simulink subsystem "PVcontroller"  (R2023a)
settings: Solver=VariableStepAuto  StartTime=0.0  StopTime=10.0  RelTol=1e-3
model mask{L=PVInverter.L, frequency=Grid.frequency, iMax=PVInverter.I_max_pu, zBase=Base.z_base, mVAbase=Base.MVA_base_new, VdcBase=PVController.Vdc_base, sampleTime=-1, Choice=Incremental conductance (INC), Vdc=PVInverter.Vdc, delV=10, tSettling=Mpp.ts, Kppll=PLL.Kp_pll, Kipll=PLL.Ki_pll, initialPhase=0, Kpv=PVController.Kp_v, Kiv=PVController.Ki_v, Kdv=0, Kpicd=PVController.Kp_ic, Kiicd=PVController.Ki_ic, Kdicd=0, Kpicq=PVController.Kp_ic, Kiicq=PVController.Ki_ic, Kdicq=0}
  mask prompts: L "AC Filter Inductance (H)"; frequency "System Frequency (Hz)"; iMax "Inverter Current Limit (PU)"; zBase "Base Impedance AC Side (Ohm)"; mVAbase "Base  Volt Amper AC side"; VdcBase "DC Bus Base Voltage (V)"; Choice "Algorithm"; Vdc "Initial VoltageFor MPPT"; delV "Voltage StepOf MPPT"; tSettling "Settling Time Of MPPT (s)"; Kppll "Proportional Gain"; Kipll "Integral Gain"; initialPhase "Initial phase angle (deg)"; Kpv "Proportional Gain"; Kiv "Integral Gain"; Kdv "Derivative Gain"; Kpicd "Daxis Proportional Gain"; Kiicd "Daxis Integral Gain"; Kdicd "D axis Derivative Gain"; Kpicq "Q axis Proportional Gain"; Kiicq "Qaxis Integral Gain"; Kdicq "Qaxis Derivative Gain"
undefined symbols (not defined in the file): Mpp, Ts
libraries: simulink x10, eeGeneralControl x4, slpidlib x3, eeTransforms x3, eeSinusoidalMeasurementV2 x1
settings Model: Creator=rajarshd  LastModifiedBy=Rajarshi

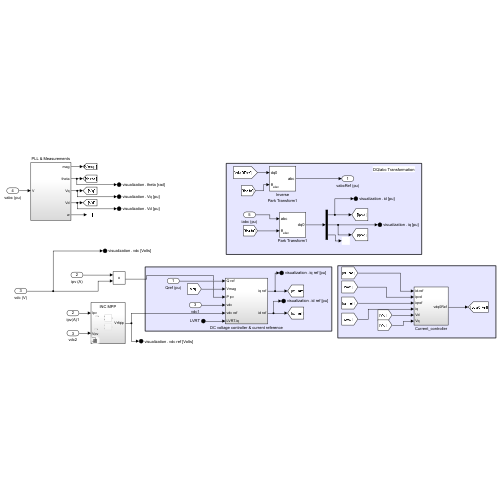
[thumbnail: Simulink's stored preview of the top-level diagram]
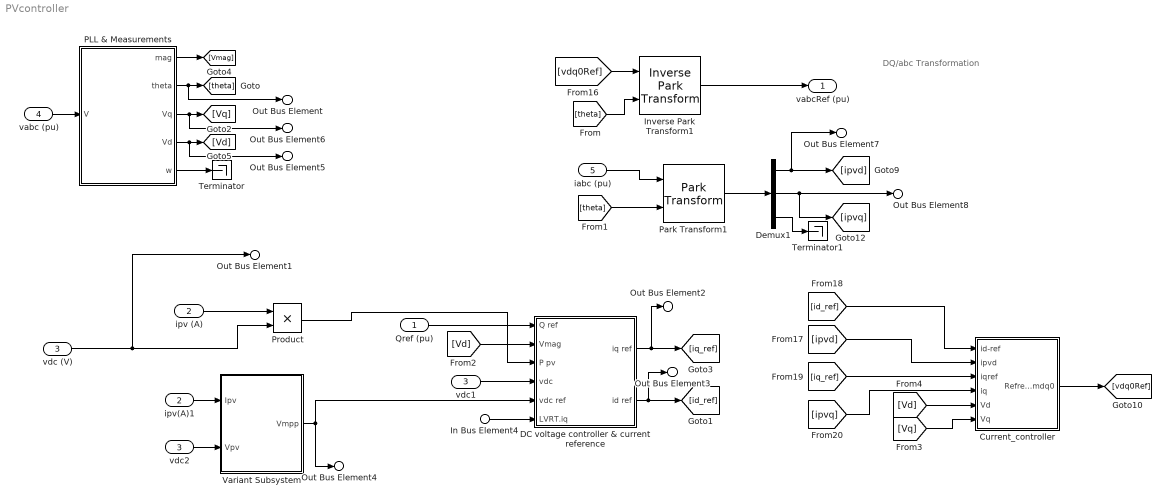
== system PVcontroller ==
  note: DQ/abc Transformation
  Qref (pu) : Inport
  ipv (A) : Inport  Port=2
  vdc (V) : Inport  Port=3
  vabc (pu) : Inport  Port=4
  iabc (pu) : Inport  Port=5
  In Bus Element4 : Inport  Port=6  PortName=LVRT
  Current_controller : Subsystem  SystemSampleTime=sampleTime
  DC voltage controller & current reference : Subsystem  SystemSampleTime=sampleTime
  Demux1 : Demux  Outputs=3
  Inverse Park Transform1 : eeTransforms/Inverse Park Transform  AxisAlignment=Q-axis  PowerInvariant=off
  PLL & Measurements : Subsystem
      settings: PortSchema="{\"entries\":[{\"content\":{\"sides\":[{\"content\":{\"connectorIds\":[\"Out1\",\"Out2\",\"Out3\",\"Out4\",\"Out5\"]},\"type\":\"ConnectorPlacement.EquallySpacedRectSide\",\"uuid\":\"76485780-20fe-4fcf-8224-69648da6ed2a\"},{\"content\":{\"connectorIds\":[\"In1\"],\"side\":\"RIGHT\"},\"type\":\"ConnectorPlacement.EquallySpacedRectSide\",\"uuid\":\"f19a6390-e634-42c7-8d46-4cd80cbab182\"},{\"content\":{\"side\":\"TOP\"},\"type\":\"ConnectorPlacement.EquallySpacedRectSide\",\"uuid\":\"87682f72-1844-428e-be70-ad7ca3191ee3\"}]},\"type\":\"ConnectorPlacement.EquallySpacedConnector\",\"uuid\":\"f2136b07-48ec-402b-adb3-18c0bac2157c\"}],\"packageUris\":[\"http://schema.mathworks.com/mf0/Connector/R2020b\"],\"version\":\"1.0\"}"
  Park Transform1 : eeTransforms/Park Transform  AxisAlignment=Q-axis  PowerInvariant=off
  Product : Product
  Terminator : Terminator
  Terminator1 : Terminator
  Variant Subsystem : Subsystem  Variant=on  VariantControlMode=label  LabelModeActiveChoice=Incremental conductance (INC)
  ipv(A)1 : InportShadow  Port=2
  vdc1 : InportShadow  Port=3
  vdc2 : InportShadow  Port=3
  vabcRef (pu) : Outport
  Out Bus Element : Outport  Port=2  PortName=visualization  Element=theta [rad]
  Out Bus Element1 : Outport  Port=2  PortName=visualization  Element=vdc [Volts]
  Out Bus Element2 : Outport  Port=2  PortName=visualization  Element=iq ref [pu]
  Out Bus Element3 : Outport  Port=2  PortName=visualization  Element=id ref [pu]
  Out Bus Element4 : Outport  Port=2  PortName=visualization  Element=vdc ref [Volts]
  Out Bus Element5 : Outport  Port=2  PortName=visualization  Element=Vd [pu]
  Out Bus Element6 : Outport  Port=2  PortName=visualization  Element=Vq [pu]
  Out Bus Element7 : Outport  Port=2  PortName=visualization  Element=id [pu]
  Out Bus Element8 : Outport  Port=2  PortName=visualization  Element=iq [pu]
  wires:
  PLL & Measurements/2(theta) -> Out Bus Element/1, [theta]
  ipv(A)1/1 -> Variant Subsystem/1(Ipv)
  vdc2/1 -> Variant Subsystem/2(Vpv)
  ipv (A)/1 -> Product/1
  PLL & Measurements/5(w) -> Terminator/1
  Variant Subsystem/1(Vmpp) -> Out Bus Element4/1, DC voltage controller & current reference/5(vdc ref)
  vdc1/1 -> DC voltage controller & current reference/4(vdc)
  vabc (pu)/1 -> PLL & Measurements/1(V)
  PLL & Measurements/4(Vd) -> Out Bus Element5/1, [Vd]
  PLL & Measurements/1(mag) -> [Vmag]
  PLL & Measurements/3(Vq) -> Out Bus Element6/1, [Vq]
  Product/1 -> DC voltage controller & current reference/3(P pv)
  vdc (V)/1 -> Out Bus Element1/1, Product/2
  Qref (pu)/1 -> DC voltage controller & current reference/1(Q ref)
  DC voltage controller & current reference/2(id ref) -> Out Bus Element3/1, [id_ref]
  DC voltage controller & current reference/1(iq ref) -> Out Bus Element2/1, [iq_ref]
  [Vd] -> DC voltage controller & current reference/2(Vmag)
  iabc (pu)/1 -> Park Transform1/1
  [ipvd] -> Current_controller/2(ipvd)
  [theta] -> Inverse Park Transform1/2
  [theta] -> Park Transform1/2
  [ipvq] -> Current_controller/4(iq)
  [iq_ref] -> Current_controller/3(iqref)
  [Vd] -> Current_controller/5(Vd)
  [id_ref] -> Current_controller/1(id-ref)
  Park Transform1/1 -> Demux1/1
  [vdq0Ref] -> Inverse Park Transform1/1
  Demux1/3 -> Terminator1/1
  Demux1/1 -> Out Bus Element7/1, [ipvd]
  Inverse Park Transform1/1 -> vabcRef (pu)/1
  Demux1/2 -> Out Bus Element8/1, [ipvq]
  Current_controller/1(Refrence_mdq0) -> [vdq0Ref]
  [Vq] -> Current_controller/6(Vq)
  In Bus Element4/1 -> DC voltage controller & current reference/6(LVRT.iq)

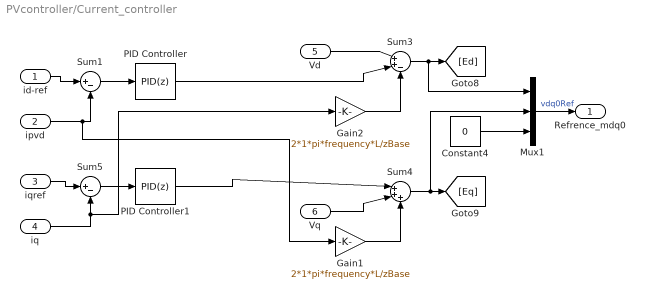
== system PVcontroller/Current_controller ==
  id-ref : Inport
  ipvd : Inport  Port=2
  iqref : Inport  Port=3
  iq : Inport  Port=4
  Vd : Inport  Port=5
  Vq : Inport  Port=6
  Constant4 : Constant  Value=0
  Gain1 : Gain  Gain=2*1*pi*frequency*L/zBase
  Gain2 : Gain  Gain=2*1*pi*frequency*L/zBase
  Mux1 : Mux  Inputs=3
  PID Controller : slpidlib/PID Controller  Controller=PID  Form=Parallel  TimeDomain=Discrete-time  UseExternalTs=off  SampleTime=-1  IntegratorMethod=Forward Euler  FilterMethod=Forward Euler  ControllerParametersSource=internal  P=Kpicd  I=Kiicd  UseKiTs=off  D=Kdicd  N=100  UseFilter=on  TunerSelectOption=Transfer Function Based (PID Tuner App)  InitialConditionSource=internal  InitialConditionForIntegrator=0  InitialConditionForFilter=0  DifferentiatorICPrevScaledInput=0  ExternalReset=none  TrackingMode=off  Kt=1  LimitOutput=off  SatLimitsSource=internal  UpperSaturationLimit=inf  LowerSaturationLimit=-inf  LinearizeAsGain=on  AntiWindupMode=clamping  Kb=1  LimitIntegrator=off  UpperIntegratorSaturationLimit=inf  LowerIntegratorSaturationLimit=-inf  POutMin=[]  POutMax=[]  IOutMin=[]  IOutMax=[]  DOutMin=[]  DOutMax=[]  NOutMin=[]  NOutMax=[]  SumOutMin=[]  SumOutMax=[]  SaturationOutMin=[]  SaturationOutMax=[]  PParamMin=[]  PParamMax=[]  IParamMin=[]  IParamMax=[]  DParamMin=[]  DParamMax=[]  NParamMin=[]  NParamMax=[]  KbParamMin=[]  KbParamMax=[]  KtParamMin=[]  KtParamMax=[]  KbOutMin=[]  KbOutMax=[]  KtOutMin=[]  KtOutMax=[]  IntegratorOutMin=[]  IntegratorOutMax=[]  FilterOutMin=[]  FilterOutMax=[]  SumI1OutMin=[]  SumI1OutMax=[]  SumI2OutMin=[]  SumI2OutMax=[]  SumI3OutMin=[]  SumI3OutMax=[]  SumI4OutMin=[]  SumI4OutMax=[]  SumDOutMin=[]  SumDOutMax=[]  DifferentiatorOutMin=[]  DifferentiatorOutMax=[]  FilterDiffOutCoefMin=[]  FilterDiffOutCoefMax=[]  ReciprocalOutMin=[]  ReciprocalOutMax=[]  SumDenOutMin=[]  SumDenOutMax=[]  SumNumOutMin=[]  SumNumOutMax=[]  DivideOutMin=[]  DivideOutMax=[]  UdiffTsProdOutMin=[]  UdiffTsProdOutMax=[]  NTsProdOutMin=[]  NTsProdOutMax=[]  UintegralTsProdOutMin=[]  UintegralTsProdOutMax=[]  UngainTsProdOutMin=[]  UngainTsProdOutMax=[]  ClampingZeroOutDataTypeStr=Inherit: Inherit via back propagation  ClampingZeroOutMin=[]  ClampingZeroOutMax=[]  FilterDenConstantOutDataTypeStr=Inherit: Inherit via back propagation  FilterDenConstantOutMin=[]  FilterDenConstantOutMax=[]  PCopyOutDataTypeStr=Inherit: Inherit via back propagation  PCopyOutMin=[]  PCopyOutMax=[]  NCopyOutDataTypeStr=Inherit: Inherit via back propagation  NCopyOutMin=[]  NCopyOutMax=[]  IntegratorContinuousStateAttributes=''  IntegratorStateMustResolveToSignalObject=off  IntegratorRTWStateStorageClass=Auto  FilterContinuousStateAttributes=''  FilterStateMustResolveToSignalObject=off  FilterRTWStateStorageClass=Auto  ParallelPVariant=InternalParameters  IdealPVariant=Disabled  IVariant=InternalParameters  DVariant=InternalParameters  IntegratorVariant=Discrete  SatVariant=Disabled  AWVariant=Passthrough  PCopyVariant=Disabled  TRVariant=Disabled  FdbkBlocksVariant=Forward  IdealPFdbkVariant=Disabled  SatFdbkVariant=Disabled  DerivativeFilterVariant=ForwardEulerFilter  NVariant=InternalParameters  NCopyVariant=Disabled  FilterICVariant=InternalICsFilter  IntegratorICVariant=InternalICs  ExternalResetVariant=Disabled  TRSumVariant=Passthrough  SumFdbkVariant=Disabled  SumVariant=Sum_PID  TsampFilterVariant=InternalTs  TsampNgainVariant=Passthrough  TsampIntegralVariant=Disabled_SignalSpec  ExternalSaturationOutDataTypeStr=Inherit: Same as second input
  PID Controller1 : slpidlib/PID Controller  Controller=PID  Form=Parallel  TimeDomain=Discrete-time  UseExternalTs=off  SampleTime=-1  IntegratorMethod=Forward Euler  FilterMethod=Forward Euler  ControllerParametersSource=internal  P=Kpicq  I=Kiicq  UseKiTs=off  D=Kdicq  N=100  UseFilter=on  TunerSelectOption=Transfer Function Based (PID Tuner App)  InitialConditionSource=internal  InitialConditionForIntegrator=0  InitialConditionForFilter=0  DifferentiatorICPrevScaledInput=0  ExternalReset=none  TrackingMode=off  Kt=1  LimitOutput=off  SatLimitsSource=internal  UpperSaturationLimit=inf  LowerSaturationLimit=-inf  LinearizeAsGain=on  AntiWindupMode=none  Kb=1  LimitIntegrator=off  UpperIntegratorSaturationLimit=inf  LowerIntegratorSaturationLimit=-inf  POutMin=[]  POutMax=[]  IOutMin=[]  IOutMax=[]  DOutMin=[]  DOutMax=[]  NOutMin=[]  NOutMax=[]  SumOutMin=[]  SumOutMax=[]  SaturationOutMin=[]  SaturationOutMax=[]  PParamMin=[]  PParamMax=[]  IParamMin=[]  IParamMax=[]  DParamMin=[]  DParamMax=[]  NParamMin=[]  NParamMax=[]  KbParamMin=[]  KbParamMax=[]  KtParamMin=[]  KtParamMax=[]  KbOutMin=[]  KbOutMax=[]  KtOutMin=[]  KtOutMax=[]  IntegratorOutMin=[]  IntegratorOutMax=[]  FilterOutMin=[]  FilterOutMax=[]  SumI1OutMin=[]  SumI1OutMax=[]  SumI2OutMin=[]  SumI2OutMax=[]  SumI3OutMin=[]  SumI3OutMax=[]  SumI4OutMin=[]  SumI4OutMax=[]  SumDOutMin=[]  SumDOutMax=[]  DifferentiatorOutMin=[]  DifferentiatorOutMax=[]  FilterDiffOutCoefMin=[]  FilterDiffOutCoefMax=[]  ReciprocalOutMin=[]  ReciprocalOutMax=[]  SumDenOutMin=[]  SumDenOutMax=[]  SumNumOutMin=[]  SumNumOutMax=[]  DivideOutMin=[]  DivideOutMax=[]  UdiffTsProdOutMin=[]  UdiffTsProdOutMax=[]  NTsProdOutMin=[]  NTsProdOutMax=[]  UintegralTsProdOutMin=[]  UintegralTsProdOutMax=[]  UngainTsProdOutMin=[]  UngainTsProdOutMax=[]  ClampingZeroOutDataTypeStr=Inherit: Inherit via back propagation  ClampingZeroOutMin=[]  ClampingZeroOutMax=[]  FilterDenConstantOutDataTypeStr=Inherit: Inherit via back propagation  FilterDenConstantOutMin=[]  FilterDenConstantOutMax=[]  PCopyOutDataTypeStr=Inherit: Inherit via back propagation  PCopyOutMin=[]  PCopyOutMax=[]  NCopyOutDataTypeStr=Inherit: Inherit via back propagation  NCopyOutMin=[]  NCopyOutMax=[]  IntegratorContinuousStateAttributes=''  IntegratorStateMustResolveToSignalObject=off  IntegratorRTWStateStorageClass=Auto  FilterContinuousStateAttributes=''  FilterStateMustResolveToSignalObject=off  FilterRTWStateStorageClass=Auto  ParallelPVariant=InternalParameters  IdealPVariant=Disabled  IVariant=InternalParameters  DVariant=InternalParameters  IntegratorVariant=Discrete  SatVariant=Disabled  AWVariant=Passthrough  PCopyVariant=Disabled  TRVariant=Disabled  FdbkBlocksVariant=Forward  IdealPFdbkVariant=Disabled  SatFdbkVariant=Disabled  DerivativeFilterVariant=ForwardEulerFilter  NVariant=InternalParameters  NCopyVariant=Disabled  FilterICVariant=InternalICsFilter  IntegratorICVariant=InternalICs  ExternalResetVariant=Disabled  TRSumVariant=Passthrough  SumFdbkVariant=Disabled  SumVariant=Sum_PID  TsampFilterVariant=InternalTs  TsampNgainVariant=Passthrough  TsampIntegralVariant=Disabled_SignalSpec  ExternalSaturationOutDataTypeStr=Inherit: Same as second input
  Sum1 : Sum  Inputs=|+-
  Sum3 : Sum  Inputs=|++-
  Sum4 : Sum  Inputs=|+++
  Sum5 : Sum  Inputs=|+-
  Refrence_mdq0 : Outport
  wires:
  PID Controller/1 -> Sum3/2
  Sum3/1 -> Mux1/1, [Ed]
  Gain2/1 -> Sum3/3
  ipvd/1 -> Gain1/1, Sum1/2
  id-ref/1 -> Sum1/1
  Gain1/1 -> Sum4/3
  Vq/1 -> Sum4/2
  iq/1 -> Gain2/1, Sum5/2
  Sum1/1 -> PID Controller/1
  Vd/1 -> Sum3/1
  Constant4/1 -> Mux1/3
  Sum5/1 -> PID Controller1/1
  iqref/1 -> Sum5/1
  PID Controller1/1 -> Sum4/1
  Sum4/1 -> Mux1/2, [Eq]
  Mux1/1 -> Refrence_mdq0/1  "vdq0Ref"

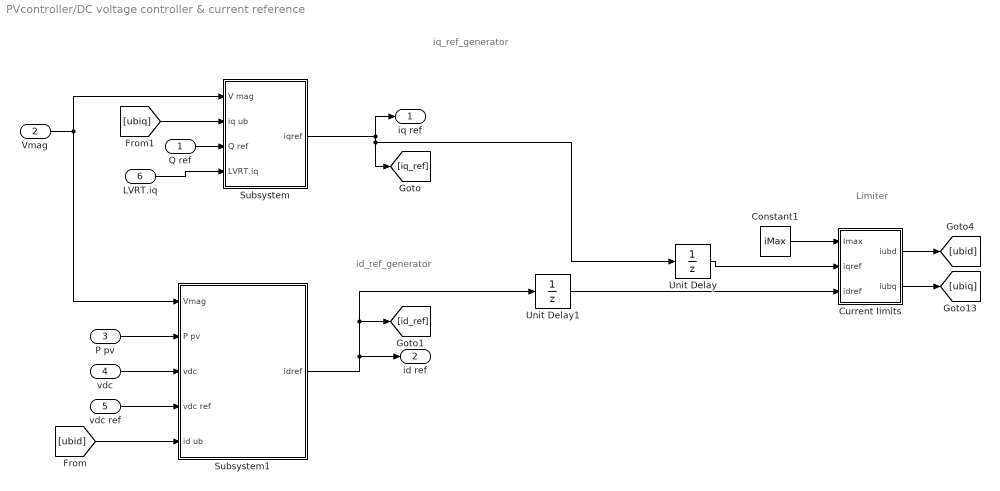
== system PVcontroller/DC voltage controller & current reference ==
  note: Limiter
  note: iq_ref_generator
  note: id_ref_generator
  Q ref : Inport
  Vmag : Inport  Port=2
  P pv : Inport  Port=3
  vdc : Inport  Port=4
  vdc ref : Inport  Port=5
  LVRT.iq : Inport  Port=6
  Constant1 : Constant  Value=iMax
  Current limits : Subsystem
  Subsystem : Subsystem
  Subsystem1 : Subsystem
  Unit Delay : UnitDelay  SampleTime=-1  HasFrameUpgradeWarning=on
  Unit Delay1 : UnitDelay  SampleTime=-1  HasFrameUpgradeWarning=on
  iq ref : Outport
  id ref : Outport  Port=2
  wires:
  Unit Delay1/1 -> Current limits/3(idref)
  Unit Delay/1 -> Current limits/2(iqref)
  LVRT.iq/1 -> Subsystem/4(LVRT.iq)
  Current limits/2(iubq) -> [ubiq]
  Current limits/1(iubd) -> [ubid]
  Constant1/1 -> Current limits/1(Imax)
  Q ref/1 -> Subsystem/3(Q ref)
  Subsystem1/1(idref) -> [id_ref], Unit Delay1/1, id ref/1
  P pv/1 -> Subsystem1/2(P pv)
  vdc/1 -> Subsystem1/3(vdc)
  vdc ref/1 -> Subsystem1/4(vdc ref)
  Subsystem/1(iqref) -> Unit Delay/1, [iq_ref], iq ref/1
  [ubid] -> Subsystem1/5(id ub)
  [ubiq] -> Subsystem/2(iq ub)
  Vmag/1 -> Subsystem1/1(Vmag), Subsystem/1(V mag)

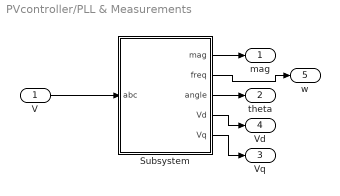
== system PVcontroller/PLL & Measurements ==
  V : Inport
  Subsystem : Subsystem
  mag : Outport
  theta : Outport  Port=2
  Vq : Outport  Port=3
  Vd : Outport  Port=4
  w : Outport  Port=5
  wires:
  V/1 -> Subsystem/1(abc)
  Subsystem/1(mag) -> mag/1
  Subsystem/3(angle) -> theta/1
  Subsystem/5(Vq) -> Vq/1
  Subsystem/4(Vd) -> Vd/1
  Subsystem/2(freq) -> w/1

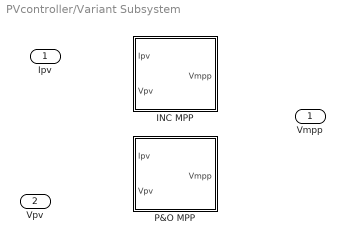
== system PVcontroller/Variant Subsystem ==
  Ipv : Inport
  Vpv : Inport  Port=2
  INC MPP : Subsystem  VariantControl=Incremental conductance (INC)
  P&O MPP : Subsystem  VariantControl=Perturb and observe (P&O)
  Vmpp : Outport

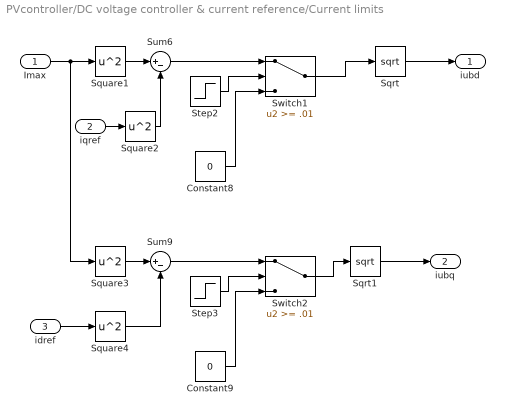
== system PVcontroller/DC voltage controller & current reference/Current limits ==
  Imax : Inport
  iqref : Inport  Port=2
  idref : Inport  Port=3
  Constant8 : Constant  Value=0
  Constant9 : Constant  Value=0
  Sqrt : Sqrt
  Sqrt1 : Sqrt
  Square{1..4} (4 alike) : Math  Operator=square
  Step2 : Step  Time=0.01  SampleTime=Ts
  Step3 : Step  Time=0.01  SampleTime=Ts
  Sum6 : Sum  Inputs=|+-
  Sum9 : Sum  Inputs=|+-
  Switch1 : Switch  Threshold=.01  SaturateOnIntegerOverflow=off  InputSameDT=off
  Switch2 : Switch  Threshold=.01  SaturateOnIntegerOverflow=off  InputSameDT=off
  iubd : Outport
  iubq : Outport  Port=2
  wires:
  idref/1 -> Square4/1
  Sqrt1/1 -> iubq/1
  Imax/1 -> Square1/1, Square3/1
  Sqrt/1 -> iubd/1
  Constant9/1 -> Switch2/3
  Square4/1 -> Sum9/2
  Constant8/1 -> Switch1/3
  Square2/1 -> Sum6/2
  Sum6/1 -> Switch1/1
  Square3/1 -> Sum9/1
  iqref/1 -> Square2/1
  Switch1/1 -> Sqrt/1
  Square1/1 -> Sum6/1
  Switch2/1 -> Sqrt1/1
  Step2/1 -> Switch1/2
  Step3/1 -> Switch2/2
  Sum9/1 -> Switch2/1

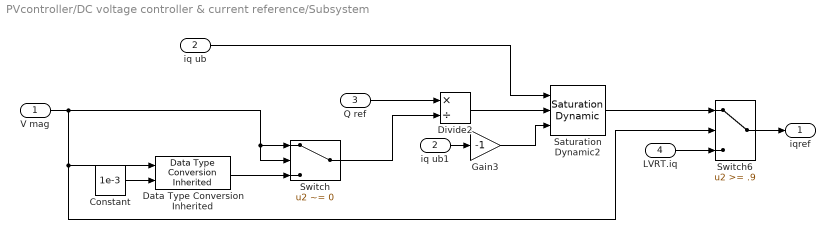
== system PVcontroller/DC voltage controller & current reference/Subsystem ==
  V mag : Inport
  iq ub : Inport  Port=2
  Q ref : Inport  Port=3
  LVRT.iq : Inport  Port=4
  Constant : Constant  Value=1e-3
  Data Type Conversion Inherited : simulink/Signal Attributes/Data Type Conversion Inherited  ConvertRealWorld=Real World Value  DoSatur=off
  Divide2 : Product  Inputs=*/
  Gain3 : Gain  Gain=-1
  Saturation Dynamic2 : simulink/Discontinuities/Saturation Dynamic  OutMin=[]  OutMax=[]  OutDataTypeStr=Inherit: Same as second input  OutDataType=fixdt(1, 16)  OutScaling=2^-10  DoSatur=off
  Switch : Switch  Criteria=u2 ~= 0  SaturateOnIntegerOverflow=off  InputSameDT=off
  Switch6 : Switch  Threshold=.9  SaturateOnIntegerOverflow=off  InputSameDT=off
  iq ub1 : InportShadow  Port=2
  iqref : Outport
  wires:
  LVRT.iq/1 -> Switch6/3
  Switch6/1 -> iqref/1
  Saturation Dynamic2/1 -> Switch6/1
  iq ub1/1 -> Gain3/1
  Divide2/1 -> Saturation Dynamic2/2
  Q ref/1 -> Divide2/1
  Gain3/1 -> Saturation Dynamic2/3
  iq ub/1 -> Saturation Dynamic2/1
  V mag/1 -> Switch/2, Switch/1, Switch6/2, Data Type Conversion Inherited/1
  Switch/1 -> Divide2/2
  Constant/1 -> Data Type Conversion Inherited/2
  Data Type Conversion Inherited/1 -> Switch/3

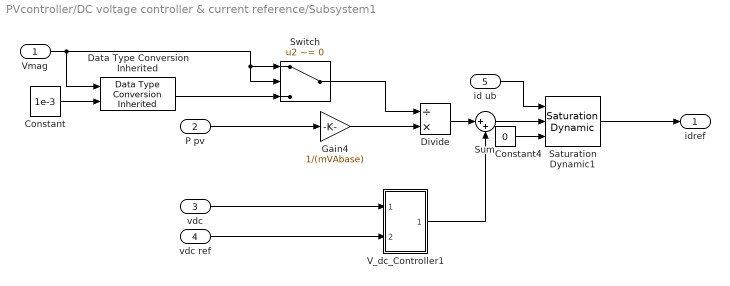
== system PVcontroller/DC voltage controller & current reference/Subsystem1 ==
  Vmag : Inport
  P pv : Inport  Port=2
  vdc : Inport  Port=3
  vdc ref : Inport  Port=4
  id ub : Inport  Port=5
  Constant : Constant  Value=1e-3
  Constant4 : Constant  Value=0
  Data Type Conversion Inherited : simulink/Signal Attributes/Data Type Conversion Inherited  ConvertRealWorld=Real World Value  DoSatur=off
  Divide : Product  Inputs=/*
  Gain4 : Gain  Gain=1/(mVAbase)
  Saturation Dynamic1 : simulink/Discontinuities/Saturation Dynamic  OutMin=[]  OutMax=[]  OutDataTypeStr=Inherit: Same as second input  OutDataType=fixdt(1, 16)  OutScaling=2^-10  DoSatur=off
  Sum : Sum  Inputs=|++
  Switch : Switch  Criteria=u2 ~= 0  SaturateOnIntegerOverflow=off  InputSameDT=off
  V_dc_Controller1 : Subsystem
  idref : Outport
  wires:
  Saturation Dynamic1/1 -> idref/1
  Constant4/1 -> Saturation Dynamic1/3
  P pv/1 -> Gain4/1
  V_dc_Controller1/1(Out1) -> Sum/2
  Sum/1 -> Saturation Dynamic1/2
  vdc ref/1 -> V_dc_Controller1/2(vdc ref)
  id ub/1 -> Saturation Dynamic1/1
  Gain4/1 -> Divide/2
  Divide/1 -> Sum/1
  vdc/1 -> V_dc_Controller1/1(vdc)
  Vmag/1 -> Data Type Conversion Inherited/1, Switch/2, Switch/1
  Switch/1 -> Divide/1
  Constant/1 -> Data Type Conversion Inherited/2
  Data Type Conversion Inherited/1 -> Switch/3

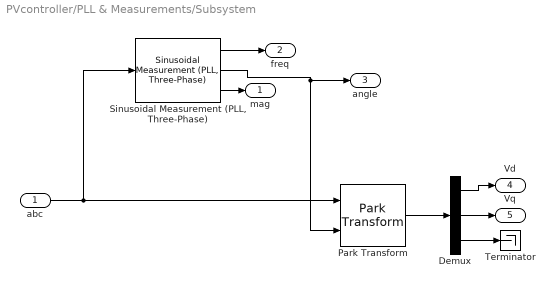
== system PVcontroller/PLL & Measurements/Subsystem ==
  abc : Inport
  Demux : Demux  Outputs=3
  Park Transform : eeTransforms/Park Transform  AxisAlignment=Q-axis  PowerInvariant=off
  "Sinusoidal Measurement (PLL, Three-Phase)" : eeSinusoidalMeasurementV2/Sinusoidal Measurement (PLL, Three-Phase)  Kp_LF=Kppll  Ki_LF=Kipll  F0=frequency  Theta0=initialPhase  Ts=sampleTime
      link override Park Transform: PowerInvariant=off
  Terminator : Terminator
  mag : Outport
  freq : Outport  Port=2
  angle : Outport  Port=3
  Vd : Outport  Port=4
  Vq : Outport  Port=5
  wires:
  Demux/3 -> Terminator/1
  abc/1 -> Park Transform/1, "Sinusoidal Measurement (PLL, Three-Phase)"/1
  Park Transform/1 -> Demux/1
  Demux/1 -> Vd/1
  Demux/2 -> Vq/1
  "Sinusoidal Measurement (PLL, Three-Phase)"/1 -> freq/1
  "Sinusoidal Measurement (PLL, Three-Phase)"/3 -> mag/1
  "Sinusoidal Measurement (PLL, Three-Phase)"/2 -> Park Transform/2, angle/1

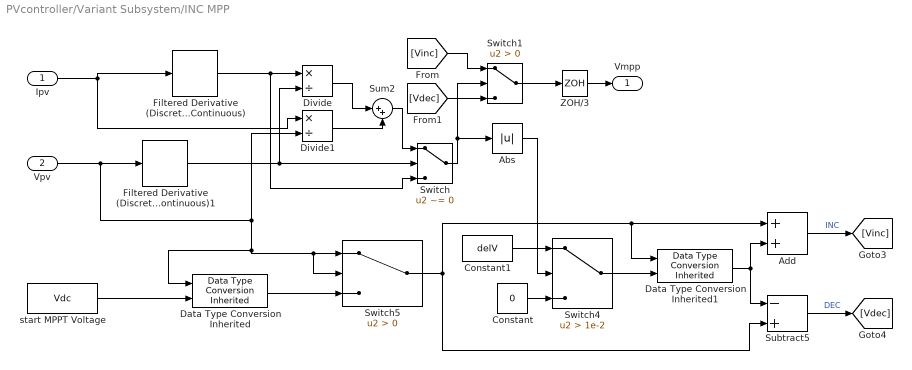
== system PVcontroller/Variant Subsystem/INC MPP ==
  Ipv : Inport
  Vpv : Inport  Port=2
  Abs : Abs  SaturateOnIntegerOverflow=off
  Add : Sum
  Constant : Constant  Value=0  SampleTime=sampleTime
  Constant1 : Constant  Value=delV  SampleTime=sampleTime
  Data Type Conversion Inherited : simulink/Signal Attributes/Data Type Conversion Inherited  ConvertRealWorld=Real World Value  DoSatur=off
  Data Type Conversion Inherited1 : simulink/Signal Attributes/Data Type Conversion Inherited  ConvertRealWorld=Real World Value  DoSatur=off
  Divide : Product  Inputs=*/
  Divide1 : Product  Inputs=*/
  Filtered Derivative (Discrete or Continuous) : eeGeneralControl/Filtered Derivative (Discrete or Continuous)  K=1  T=tSettling*2  B=inf  A=-inf  minRatio=1  init_option=Inherited from block input  x0=0  Ts=sampleTime
      settings: LibrarySourceBlock=|
      | ee_sl_lib/General Control/Filtered Derivative
      | (Discrete or Continuous)
  Filtered Derivative (Discrete or Continuous)1 : eeGeneralControl/Filtered Derivative (Discrete or Continuous)  K=1  T=tSettling*2  B=inf  A=-inf  minRatio=1  init_option=Inherited from block input  x0=0  Ts=sampleTime
      settings: LibrarySourceBlock=|
      | ee_sl_lib/General Control/Filtered Derivative
      | (Discrete or Continuous)
  Subtract5 : Sum  Inputs=-+
  Sum2 : Sum  Inputs=|++
  Switch : Switch  Criteria=u2 ~= 0  SaturateOnIntegerOverflow=off  InputSameDT=off
  Switch1 : Switch  Criteria=u2 > Threshold  SaturateOnIntegerOverflow=off  InputSameDT=off
  Switch4 : Switch  Criteria=u2 > Threshold  Threshold=1e-2  SaturateOnIntegerOverflow=off  InputSameDT=off
  Switch5 : Switch  Criteria=u2 > Threshold  SaturateOnIntegerOverflow=off  InputSameDT=off
  ZOH/3 : ZeroOrderHold  SampleTime=Mpp.td
  start MPPT Voltage : Constant  Value=Vdc  SampleTime=sampleTime
  Vmpp : Outport  VectorParamsAs1DForOutWhenUnconnected=off
  wires:
  ZOH/3/1 -> Vmpp/1
  Ipv/1 -> Filtered Derivative (Discrete or Continuous)/1, Divide1/1
  Switch5/1 -> Data Type Conversion Inherited1/1, Add/1, Subtract5/2
  Vpv/1 -> Filtered Derivative (Discrete or Continuous)1/1, Divide1/2, Data Type Conversion Inherited/1, Switch5/2, Switch5/1
  Add/1 -> [Vinc]  "INC"
  Subtract5/1 -> [Vdec]  "DEC"
  Filtered Derivative (Discrete or Continuous)/1 -> Switch/3, Divide/1
  Divide/1 -> Sum2/1
  Divide1/1 -> Sum2/2
  Sum2/1 -> Switch/1
  Switch/1 -> Switch1/2, Abs/1
  [Vinc] -> Switch1/1
  [Vdec] -> Switch1/3
  Filtered Derivative (Discrete or Continuous)1/1 -> Switch/2, Divide/2
  Abs/1 -> Switch4/2
  Constant/1 -> Switch4/3
  Constant1/1 -> Switch4/1
  Switch1/1 -> ZOH/3/1
  Data Type Conversion Inherited/1 -> Switch5/3
  start MPPT Voltage/1 -> Data Type Conversion Inherited/2
  Switch4/1 -> Data Type Conversion Inherited1/2
  Data Type Conversion Inherited1/1 -> Add/2, Subtract5/1

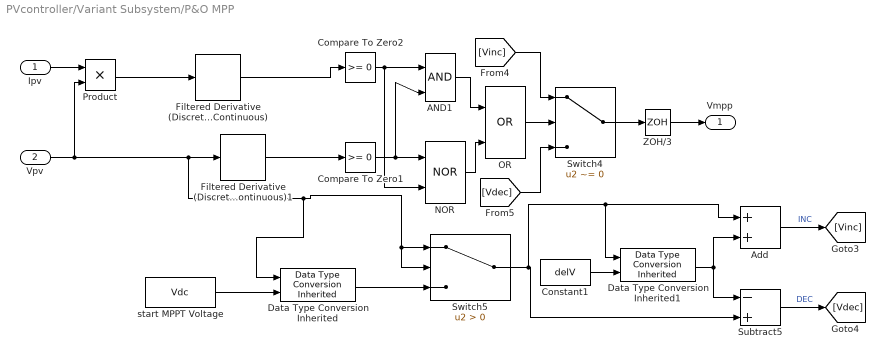
== system PVcontroller/Variant Subsystem/P&O MPP ==
  Ipv : Inport
  Vpv : Inport  Port=2
  AND1 : Logic  IconShape=distinctive  AllPortsSameDT=off  OutDataTypeStr=boolean
  Add : Sum
  Compare To Zero1 : simulink/Logic and Bit Operations/Compare To Zero  relop=>=  OutDataTypeStr=boolean
  Compare To Zero2 : simulink/Logic and Bit Operations/Compare To Zero  relop=>=  OutDataTypeStr=boolean
  Constant1 : Constant  Value=delV  SampleTime=sampleTime
  Data Type Conversion Inherited : simulink/Signal Attributes/Data Type Conversion Inherited  ConvertRealWorld=Real World Value  DoSatur=off
  Data Type Conversion Inherited1 : simulink/Signal Attributes/Data Type Conversion Inherited  ConvertRealWorld=Real World Value  DoSatur=off
  Filtered Derivative (Discrete or Continuous) : eeGeneralControl/Filtered Derivative (Discrete or Continuous)  K=1  T=tSettling*2  B=inf  A=-inf  minRatio=1  init_option=Inherited from block input  x0=0  Ts=sampleTime
      settings: LibrarySourceBlock=|
      | ee_sl_lib/General Control/Filtered Derivative
      | (Discrete or Continuous)
  Filtered Derivative (Discrete or Continuous)1 : eeGeneralControl/Filtered Derivative (Discrete or Continuous)  K=1  T=tSettling*2  B=inf  A=-inf  minRatio=1  init_option=Inherited from block input  x0=0  Ts=sampleTime
      settings: LibrarySourceBlock=|
      | ee_sl_lib/General Control/Filtered Derivative
      | (Discrete or Continuous)
  NOR : Logic  Operator=NOR  IconShape=distinctive  AllPortsSameDT=off  OutDataTypeStr=boolean
  OR : Logic  Operator=OR  IconShape=distinctive  AllPortsSameDT=off  OutDataTypeStr=boolean
  Product : Product
  Subtract5 : Sum  Inputs=-+
  Switch4 : Switch  Criteria=u2 ~= 0  SaturateOnIntegerOverflow=off  InputSameDT=off
  Switch5 : Switch  Criteria=u2 > Threshold  SaturateOnIntegerOverflow=off  InputSameDT=off
  ZOH/3 : ZeroOrderHold  SampleTime=Mpp.td
  start MPPT Voltage : Constant  Value=Vdc  SampleTime=sampleTime
  Vmpp : Outport  VectorParamsAs1DForOutWhenUnconnected=off
  wires:
  ZOH/3/1 -> Vmpp/1
  OR/1 -> Switch4/2
  Compare To Zero1/1 -> NOR/1, AND1/2
  Compare To Zero2/1 -> NOR/2, AND1/1
  Switch5/1 -> Data Type Conversion Inherited1/1, Add/1, Subtract5/2
  Constant1/1 -> Data Type Conversion Inherited1/2
  Vpv/1 -> Product/2, Filtered Derivative (Discrete or Continuous)1/1, Data Type Conversion Inherited/1, Switch5/2, Switch5/1
  Add/1 -> [Vinc]  "INC"
  NOR/1 -> OR/2
  Subtract5/1 -> [Vdec]  "DEC"
  [Vdec] -> Switch4/3
  Filtered Derivative (Discrete or Continuous)1/1 -> Compare To Zero1/1
  Filtered Derivative (Discrete or Continuous)/1 -> Compare To Zero2/1
  AND1/1 -> OR/1
  [Vinc] -> Switch4/1
  Ipv/1 -> Product/1
  Product/1 -> Filtered Derivative (Discrete or Continuous)/1
  Switch4/1 -> ZOH/3/1
  Data Type Conversion Inherited/1 -> Switch5/3
  start MPPT Voltage/1 -> Data Type Conversion Inherited/2
  Data Type Conversion Inherited1/1 -> Add/2, Subtract5/1

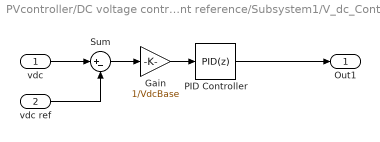
== system PVcontroller/DC voltage controller & current reference/Subsystem1/V_dc_Controller1 ==
  vdc : Inport
  vdc ref : Inport  Port=2
  Gain : Gain  Gain=1/VdcBase
  PID Controller : slpidlib/PID Controller  Controller=PID  Form=Parallel  TimeDomain=Discrete-time  UseExternalTs=off  SampleTime=-1  IntegratorMethod=Forward Euler  FilterMethod=Forward Euler  ControllerParametersSource=internal  P=Kpv  I=Kiv  UseKiTs=off  D=Kdv  N=100  UseFilter=on  TunerSelectOption=Transfer Function Based (PID Tuner App)  ZeroCross=off  InitialConditionSource=internal  InitialConditionForIntegrator=0  InitialConditionForFilter=0  DifferentiatorICPrevScaledInput=0  ExternalReset=none  TrackingMode=off  Kt=1  LimitOutput=off  SatLimitsSource=internal  UpperSaturationLimit=iMax  LowerSaturationLimit=0  LinearizeAsGain=on  AntiWindupMode=clamping  Kb=1  LimitIntegrator=off  UpperIntegratorSaturationLimit=inf  LowerIntegratorSaturationLimit=-inf  POutMin=[]  POutMax=[]  IOutMin=[]  IOutMax=[]  DOutMin=[]  DOutMax=[]  NOutMin=[]  NOutMax=[]  SumOutMin=[]  SumOutMax=[]  SaturationOutMin=[]  SaturationOutMax=[]  PParamMin=[]  PParamMax=[]  IParamMin=[]  IParamMax=[]  DParamMin=[]  DParamMax=[]  NParamMin=[]  NParamMax=[]  KbParamMin=[]  KbParamMax=[]  KtParamMin=[]  KtParamMax=[]  KbOutMin=[]  KbOutMax=[]  KtOutMin=[]  KtOutMax=[]  IntegratorOutMin=[]  IntegratorOutMax=[]  FilterOutMin=[]  FilterOutMax=[]  SumI1OutMin=[]  SumI1OutMax=[]  SumI2OutMin=[]  SumI2OutMax=[]  SumI3OutMin=[]  SumI3OutMax=[]  SumI4OutMin=[]  SumI4OutMax=[]  SumDOutMin=[]  SumDOutMax=[]  DifferentiatorOutMin=[]  DifferentiatorOutMax=[]  FilterDiffOutCoefMin=[]  FilterDiffOutCoefMax=[]  ReciprocalOutMin=[]  ReciprocalOutMax=[]  SumDenOutMin=[]  SumDenOutMax=[]  SumNumOutMin=[]  SumNumOutMax=[]  DivideOutMin=[]  DivideOutMax=[]  UdiffTsProdOutMin=[]  UdiffTsProdOutMax=[]  NTsProdOutMin=[]  NTsProdOutMax=[]  UintegralTsProdOutMin=[]  UintegralTsProdOutMax=[]  UngainTsProdOutMin=[]  UngainTsProdOutMax=[]  ClampingZeroOutDataTypeStr=Inherit: Inherit via back propagation  ClampingZeroOutMin=[]  ClampingZeroOutMax=[]  FilterDenConstantOutDataTypeStr=Inherit: Inherit via back propagation  FilterDenConstantOutMin=[]  FilterDenConstantOutMax=[]  PCopyOutDataTypeStr=Inherit: Inherit via back propagation  PCopyOutMin=[]  PCopyOutMax=[]  NCopyOutDataTypeStr=Inherit: Inherit via back propagation  NCopyOutMin=[]  NCopyOutMax=[]  IntegratorContinuousStateAttributes=''  IntegratorStateMustResolveToSignalObject=off  IntegratorRTWStateStorageClass=Auto  FilterContinuousStateAttributes=''  FilterStateMustResolveToSignalObject=off  FilterRTWStateStorageClass=Auto  ParallelPVariant=InternalParameters  IdealPVariant=Disabled  IVariant=InternalParameters  DVariant=InternalParameters  IntegratorVariant=Discrete  SatVariant=Disabled  AWVariant=Passthrough  PCopyVariant=Disabled  TRVariant=Disabled  FdbkBlocksVariant=Forward  IdealPFdbkVariant=Disabled  SatFdbkVariant=Disabled  DerivativeFilterVariant=ForwardEulerFilter  NVariant=InternalParameters  NCopyVariant=Disabled  FilterICVariant=InternalICsFilter  IntegratorICVariant=InternalICs  ExternalResetVariant=Disabled  TRSumVariant=Passthrough  SumFdbkVariant=Disabled  SumVariant=Sum_PID  TsampFilterVariant=InternalTs  TsampNgainVariant=Passthrough  TsampIntegralVariant=Disabled_SignalSpec  ExternalSaturationOutDataTypeStr=Inherit: Same as second input
  Sum : Sum  Inputs=|+-
  Out1 : Outport
  wires:
  vdc/1 -> Sum/1
  vdc ref/1 -> Sum/2
  PID Controller/1 -> Out1/1
  Gain/1 -> PID Controller/1
  Sum/1 -> Gain/1
